simulink model "Sim_Q9"  (R2023b)
settings: Solver=VariableStepAuto  StartTime=-0.5  StopTime=2.0  RelTol=1e-3
settings Model: Creator=lucas  LastModifiedBy=Lucas

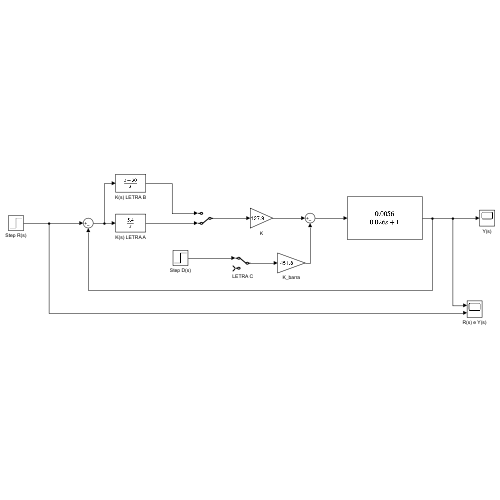
[thumbnail: Simulink's stored preview of the top-level diagram]
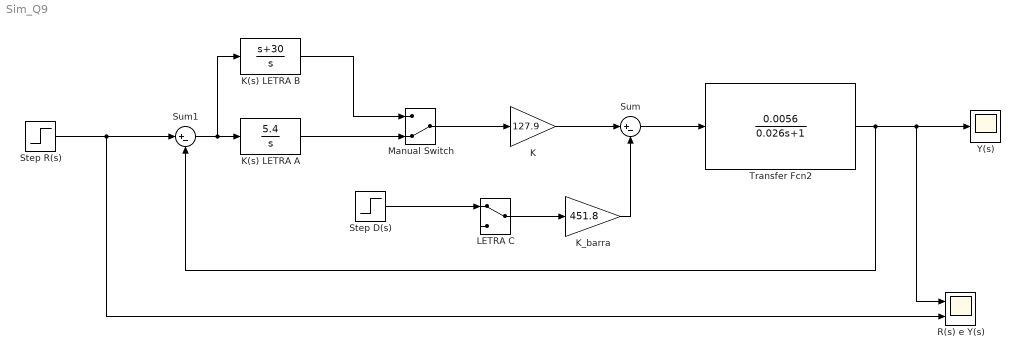
== system Sim_Q9 ==
  K : Gain  Gain=127.9
  K(s) LETRA A : TransferFcn  Numerator=[5.4]  Denominator=[1 0]
  K(s) LETRA B : TransferFcn  Numerator=[1 30]  Denominator=[1 0]
  K_barra : Gain  Gain=451.8
  LETRA C : ManualSwitch
  Manual Switch : ManualSwitch  CurrentSetting=0
  R(s) e Y(s) : Scope  NumInputPorts=2
  Step D(s) : Step  After=0.2  SampleTime=0
  Step R(s) : Step  Time=0  After=12  SampleTime=0
  Sum : Sum  Inputs=|+-
  Sum1 : Sum  Inputs=|+-
  Transfer Fcn2 : TransferFcn  Numerator=[0.0056]  Denominator=[0.026 1]
  Y(s) : Scope
  wires:
  K/1 -> Sum/1
  K(s) LETRA A/1 -> Manual Switch/2
  Sum1/1 -> K(s) LETRA B/1, K(s) LETRA A/1
  K(s) LETRA B/1 -> Manual Switch/1
  Manual Switch/1 -> K/1
  Step R(s)/1 -> R(s) e Y(s)/2, Sum1/1
  Sum/1 -> Transfer Fcn2/1
  Transfer Fcn2/1 -> Sum1/2, R(s) e Y(s)/1, Y(s)/1
  K_barra/1 -> Sum/2
  LETRA C/1 -> K_barra/1
  Step D(s)/1 -> LETRA C/1
